simulink model "nasaBatterysim"  (R2019a)
settings: Solver=FixedStepAuto  StartTime=0.0  StopTime=64.5  FixedStep=.01  RelTol=1e-3
settings Model: Creator=tdarrah  LastModifiedBy=tdarrah
settings DebuggingCC: ArithmeticOperatorsInVariantConditions=warning

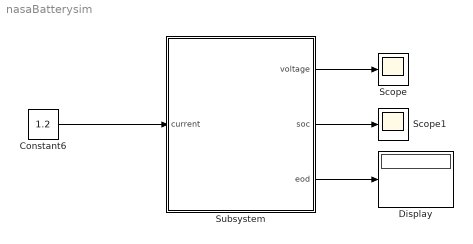
== system nasaBatterysim ==
  Constant6 : Constant  Value=1.2
  Display : Display
  Scope : Scope
  Scope1 : Scope
  Subsystem : Subsystem
  wires:
  Constant6/1 -> Subsystem/1(current)
  Subsystem/1(voltage) -> Scope/1
  Subsystem/2(soc) -> Scope1/1
  Subsystem/3(eod) -> Display/1

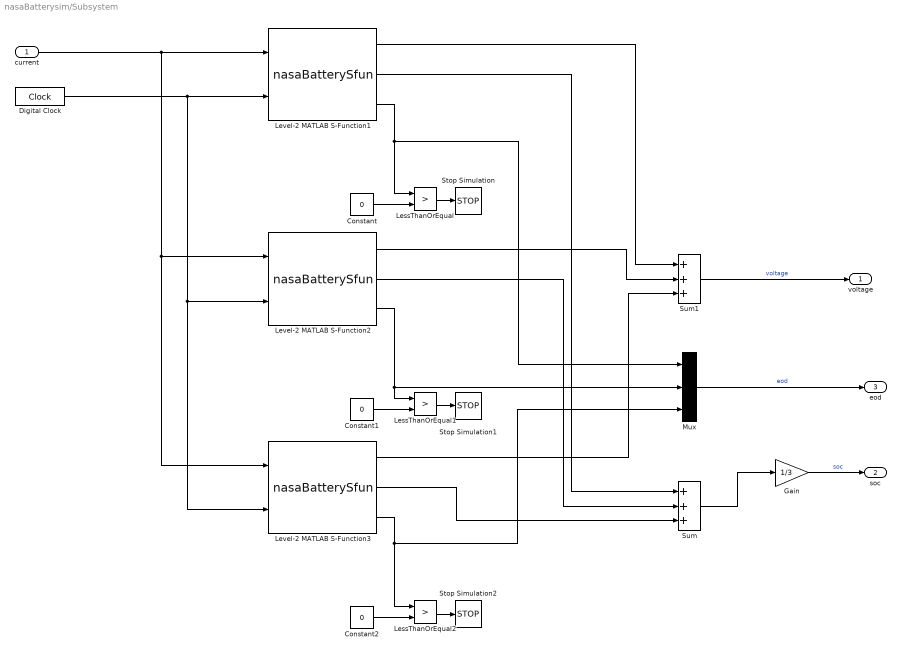
== system nasaBatterysim/Subsystem ==
  current : Inport
  Constant : Constant  Value=0
  Constant1 : Constant  Value=0
  Constant2 : Constant  Value=0
  Digital Clock : DigitalClock
      mask Display: disp('simTime');
  Gain : Gain  Gain=1/3
  LessThanOrEqual : RelationalOperator  Operator=>  OutDataTypeStr=boolean  RndMeth=Simplest
  LessThanOrEqual1 : RelationalOperator  Operator=>  OutDataTypeStr=boolean  RndMeth=Simplest
  LessThanOrEqual2 : RelationalOperator  Operator=>  OutDataTypeStr=boolean  RndMeth=Simplest
  Level-2 MATLAB S-Function1 : M-S-Function  FunctionName=nasaBatterySfun  Parameters=batteryParams
      mask Display:
      | port_label('input', 1, 'current');
      | port_label('input', 2, 'simTime');
      | port_label('output', 1, 'voltage');
      | port_label('output', 2, 'soc');
      | port_label('output', 3, 'eod');
  Level-2 MATLAB S-Function2 : M-S-Function  FunctionName=nasaBatterySfun  Parameters=batteryParams
      mask Display:
      | port_label('input', 1, 'current');
      | port_label('input', 2, 'simTime');
      | port_label('output', 1, 'voltage');
      | port_label('output', 2, 'soc');
      | port_label('output', 3, 'eod');
  Level-2 MATLAB S-Function3 : M-S-Function  FunctionName=nasaBatterySfun  Parameters=batteryParams
      mask Display:
      | port_label('input', 1, 'current');
      | port_label('input', 2, 'simTime');
      | port_label('output', 1, 'voltage');
      | port_label('output', 2, 'soc');
      | port_label('output', 3, 'eod');
  Mux : Mux  Inputs=3
  Stop Simulation : Stop
  Stop Simulation1 : Stop
  Stop Simulation2 : Stop
  Sum : Sum  Inputs=+++
  Sum1 : Sum  Inputs=+++
  voltage : Outport
  soc : Outport  Port=2
  eod : Outport  Port=3
  wires:
  Level-2 MATLAB S-Function1/1 -> Sum1/1
  Level-2 MATLAB S-Function2/1 -> Sum1/2
  LessThanOrEqual2/1 -> Stop Simulation2/1
  Constant/1 -> LessThanOrEqual/2
  LessThanOrEqual/1 -> Stop Simulation/1
  Constant2/1 -> LessThanOrEqual2/2
  Level-2 MATLAB S-Function3/1 -> Sum1/3
  Constant1/1 -> LessThanOrEqual1/2
  Mux/1 -> eod/1  "eod"
  Level-2 MATLAB S-Function3/3 -> LessThanOrEqual2/1, Mux/3
  LessThanOrEqual1/1 -> Stop Simulation1/1
  current/1 -> Level-2 MATLAB S-Function3/1, Level-2 MATLAB S-Function2/1, Level-2 MATLAB S-Function1/1
  Level-2 MATLAB S-Function2/2 -> Sum/2
  Level-2 MATLAB S-Function3/2 -> Sum/3
  Sum/1 -> Gain/1
  Gain/1 -> soc/1  "soc"
  Digital Clock/1 -> Level-2 MATLAB S-Function3/2, Level-2 MATLAB S-Function2/2, Level-2 MATLAB S-Function1/2
  Level-2 MATLAB S-Function2/3 -> Mux/2, LessThanOrEqual1/1
  Level-2 MATLAB S-Function1/3 -> Mux/1, LessThanOrEqual/1
  Sum1/1 -> voltage/1  "voltage"
  Level-2 MATLAB S-Function1/2 -> Sum/1
